simulink library "twoNodeTether_cl"  (R2018b)
settings: Solver=VariableStepAuto  StartTime=0.0  StopTime=10.0  RelTol=1e-3
libraries: nodeDragForce_ul x1, nodeNetBuoyForce_ul x1, nodeSpringDamperForce_ul x1
settings Model: Creator=mcobb  LastModifiedBy=asiddiq2

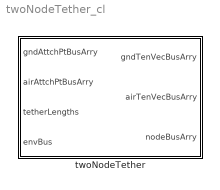
== system twoNodeTether_cl ==
  twoNodeTether : Subsystem  mask{thr=0, flowDensity=10, gravity=0}
      mask prompts: thr "Tether Structure"; flowDensity "Fluid Density"; gravity "Gravitational Acceleration"

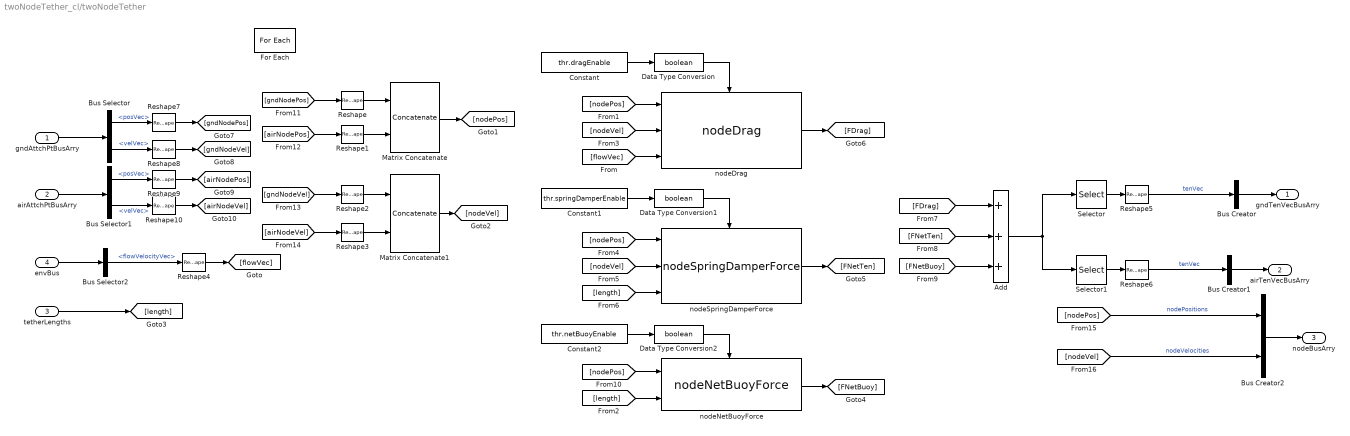
== system twoNodeTether_cl/twoNodeTether ==
  gndAttchPtBusArry : Inport  OutDataTypeStr=Bus: thrAttachPtKinematicsBus  Partition=on  PartitionDimension=1  PartitionWidth=1  PartitionOffset=0
  airAttchPtBusArry : Inport  Port=2  OutDataTypeStr=Bus: thrAttachPtKinematicsBus  Partition=on  PartitionDimension=1  PartitionWidth=1  PartitionOffset=0
  tetherLengths : Inport  Port=3  Partition=on  PartitionDimension=1  PartitionWidth=1  PartitionOffset=0
  envBus : Inport  Port=4  OutDataTypeStr=Bus: envBus
  Add : Sum  Inputs=3
  Bus Creator : BusCreator  Inputs=1  OutDataTypeStr=Bus: thrTenVecBus  NonVirtualBus=on
  Bus Creator1 : BusCreator  Inputs=1  OutDataTypeStr=Bus: thrTenVecBus  NonVirtualBus=on
  Bus Creator2 : BusCreator  Inputs=2  OutDataTypeStr=Bus: thrNodeBus  NonVirtualBus=on
  Bus Selector : BusSelector  OutputSignals=posVec,velVec
  Bus Selector1 : BusSelector  OutputSignals=posVec,velVec
  Bus Selector2 : BusSelector  OutputSignals=flowVelocityVec
  Constant : Constant  Value=thr.dragEnable
  Constant1 : Constant  Value=thr.springDamperEnable
  Constant2 : Constant  Value=thr.netBuoyEnable
  Data Type Conversion : DataTypeConversion  OutDataTypeStr=boolean
  Data Type Conversion1 : DataTypeConversion  OutDataTypeStr=boolean
  Data Type Conversion2 : DataTypeConversion  OutDataTypeStr=boolean
  For Each : ForEach  DisableCoverage=on  IterateSubsysMaskParameter=on,off,off  SubsysMaskParameterIterationDimension=2,1,1  IndexMode=One-based
  Matrix Concatenate : Concatenate  Mode=Multidimensional array  ConcatenateDimension=2
  Matrix Concatenate1 : Concatenate  Mode=Multidimensional array  ConcatenateDimension=2
  Reshape{,1..10} (11 alike) : Reshape  OutputDimensionality=Column vector (2-D)
  Selector : Selector  NumberOfDimensions=2  InputPortWidth=3  IndexOptions=Select all,Index vector (dialog)  Indices=[1 3],1  OutputSizes=1,1
  Selector1 : Selector  NumberOfDimensions=2  InputPortWidth=3  IndexOptions=Select all,Index vector (dialog)  Indices=[1 3],2  OutputSizes=1,1
  nodeDrag : nodeDragForce_ul/nodeDrag  flowDensity=flowDensity  thrDiam=thr.diameter  dragCoeff=thr.dragCoeff
  nodeNetBuoyForce : nodeNetBuoyForce_ul/nodeNetBuoyForce  fluidDensity=flowDensity  tetherDensity=thr.density  diameter=thr.diameter  gravity=gravity
  nodeSpringDamperForce : nodeSpringDamperForce_ul/nodeSpringDamperForce  mass=thr.vehicleMass  zeta=thr.dampingRatio  diameter=thr.diameter  youngsMod=thr.youngsMod
  gndTenVecBusArry : Outport  ConcatenationDimension=1
  airTenVecBusArry : Outport  Port=2  ConcatenationDimension=1
  nodeBusArry : Outport  Port=3  ConcatenationDimension=1
  wires:
  [gndNodePos] -> Reshape/1
  [gndNodeVel] -> Reshape2/1
  [airNodePos] -> Reshape1/1
  [airNodeVel] -> Reshape3/1
  Reshape/1 -> Matrix Concatenate/1
  Reshape1/1 -> Matrix Concatenate/2
  Reshape3/1 -> Matrix Concatenate1/2
  Reshape2/1 -> Matrix Concatenate1/1
  Reshape4/1 -> [flowVec]
  [flowVec] -> nodeDrag/3
  Matrix Concatenate/1 -> [nodePos]
  [nodePos] -> nodeDrag/1
  tetherLengths/1 -> [length]
  [length] -> nodeNetBuoyForce/2
  [nodeVel] -> nodeDrag/2
  [nodeVel] -> nodeSpringDamperForce/2
  [nodePos] -> nodeSpringDamperForce/1
  [length] -> nodeSpringDamperForce/3
  nodeNetBuoyForce/1 -> [FNetBuoy]
  nodeSpringDamperForce/1 -> [FNetTen]
  nodeDrag/1 -> [FDrag]
  [FNetTen] -> Add/2
  [FDrag] -> Add/1
  [FNetBuoy] -> Add/3
  Selector/1 -> Reshape5/1
  Add/1 -> Selector1/1, Selector/1
  Selector1/1 -> Reshape6/1
  Reshape5/1 -> Bus Creator/1  "tenVec"
  Reshape6/1 -> Bus Creator1/1  "tenVec"
  [nodePos] -> nodeNetBuoyForce/1
  Matrix Concatenate1/1 -> [nodeVel]
  Bus Selector/1 -> Reshape7/1  "<posVec>"
  gndAttchPtBusArry/1 -> Bus Selector/1
  Bus Selector/2 -> Reshape8/1  "<velVec>"
  Bus Selector1/2 -> Reshape10/1  "<velVec>"
  airAttchPtBusArry/1 -> Bus Selector1/1
  Bus Selector1/1 -> Reshape9/1  "<posVec>"
  envBus/1 -> Bus Selector2/1
  Bus Selector2/1 -> Reshape4/1  "<flowVelocityVec>"
  Reshape7/1 -> [gndNodePos]
  Reshape8/1 -> [gndNodeVel]
  Reshape9/1 -> [airNodePos]
  Reshape10/1 -> [airNodeVel]
  Bus Creator1/1 -> airTenVecBusArry/1
  Bus Creator/1 -> gndTenVecBusArry/1
  Bus Creator2/1 -> nodeBusArry/1
  [nodePos] -> Bus Creator2/1  "nodePositions"
  [nodeVel] -> Bus Creator2/2  "nodeVelocities"
  Constant/1 -> Data Type Conversion/1
  Data Type Conversion/1 -> nodeDrag/Enable
  Data Type Conversion1/1 -> nodeSpringDamperForce/Enable
  Constant1/1 -> Data Type Conversion1/1
  Constant2/1 -> Data Type Conversion2/1
  Data Type Conversion2/1 -> nodeNetBuoyForce/Enable
